simulink library "tqd"  (R2021b)
settings: Solver=VariableStepAuto  StartTime=0.0  StopTime=10.0  RelTol=1e-3
undefined symbols (not defined in the file or in its folder): ATQD_AccelLimitInRange_X_rpm, ATQD_AccelLimitInRange_Y_Nm, ATQD_AccelLimitOvrKi_X_Nm, ATQD_AccelLimitOvrKp_X_Nm, ATQD_BOSMapD_X_rpm, ATQD_BOSMapD_Y_pct, ATQD_BOSMapR_X_rpm, ATQD_BOSMapR_Y_pct, ATQD_HVBCurrSmooth_X_A, ATQD_LHMTqMapDLC_X_rpm, ATQD_LHMTqMapDLC_Y_pct, ATQD_LHMTqMapRLC_X_rpm, ATQD_LHMTqMapRLC_Y_pct, ATQD_NormalMapDLC_X_rpm, ATQD_NormalMapDLC_Y_pct, ATQD_NormalTqDecSR_X_rpm, ATQD_NormalTqDecSR_Y_Nm, ATQD_NormalTqIncSR_X_rpm, ATQD_NormalTqIncSR_Y_Nm, ATQD_OPDMapRLC_X_rpm, ATQD_OPDMapRLC_Y_pct, ATQD_RollRegTorReq_X_rpm, ATQD_RollRegTorReq_Y_enum, ATQD_VehSpdLimitInRange_X_rpm, ATQD_VehSpdLimitInRange_Y_Nm, ATQD_VehSpdLimitOvrKi_X_Nm, ATQD_VehSpdLimitOvrKp_X_Nm, EIGHT_INT, ENUM_BRAKEPEDAL_PRESSED, ENUM_BRAKEPEDAL_RELEASED, ENUM_COMBOKEY_DOWN, ENUM_COMBOKEY_M1, ENUM_COMBOKEY_M2, ENUM_COMBOKEY_NONE, ENUM_COMBOKEY_RKNEE, ENUM_COMBOKEY_STOPLV, ENUM_COMBOKEY_UP, ENUM_CP2VKNEEREQ_REQUEST, ENUM_CP2VNLVREQ_LEVEL1, ENUM_CP2VNLVREQ_LEVEL2, ENUM_CP2VNLVREQ_LOWER, ENUM_CP2VNLVREQ_STOPLV, ENUM_CP2VNLVREQ_UPPER, ENUM_CREEPIND_DISABLE, ENUM_CREEPIND_READY, ENUM_CREEPIND_RUNNING, ENUM_CREEPIND_WARNING, ENUM_DRIVELINERELEASE_RELEASE, ENUM_EBSTORQUERWQ_LIMIT, ENUM_EBSTORQUERWQ_TORQUE, ENUM_ECPVCUDRM_CONFORT, ENUM_ECPVCUDRM_ECO, ENUM_ECPVCUDRM_NORMAL, ENUM_ECPVCUDRM_NOTAVAILABLE, ENUM_EMTqModeDrvBrk_Accel, ENUM_EMTqModeDrvBrk_Brake, ENUM_EMTqModeDrvBrk_Coast, ENUM_ETC2ACTDRIVEDIR_BACKWARD, ENUM_ETC2ACTDRIVEDIR_FORWARD, ENUM_ETC2ACTDRIVEDIR_STILL ... (+341)
libraries: simulink x109, hcu_lib x67
(part 10 of 13)

== system tqd/TQD/Input_Convert/Input Signal Convert/Big Mike Combo V2 /Combo Key Detection/Function1 Alcohol Lock/Key8 ==
  VTQD_ComboKeyCMD_enum : Inport
  VTQD_ComboKeyEn_flg : Inport  Port=2
  VTQD_ComboKeyReset_flg : Inport  Port=3
  VTQD_ComboKey7_enum : Inport  Port=4
  AND : Logic  Inputs=4  AllPortsSameDT=off  OutDataTypeStr=boolean
  Constant1 : Constant  Value=KTQD_Function1Off8_enum
  Constant2 : Constant  Value=ENUM_COMBOKEY_NONE
  Constant3 : Constant  Value=ENUM_COMBOKEY_NONE
  Constant4 : Constant  Value=ENUM_COMBOKEY_NONE
  Data Type Conversion : DataTypeConversion  OutDataTypeStr=uint8
  Delay : Delay  DelayLength=1  InitialCondition=uint8(0)
      settings: AttributesFormatString=%<InitialCondition>
  Delay1 : Delay  DelayLength=1  InitialCondition=uint8(0)
      settings: AttributesFormatString=%<InitialCondition>
  Delay2 : Delay  DelayLength=1  InitialCondition=uint8(0)
      settings: AttributesFormatString=%<InitialCondition>
  Detect Change : simulink/Logic and Bit Operations/Detect Change  vinit=boolean(0)  OutDataTypeStr=boolean
  Detect Increase : simulink/Logic and Bit Operations/Detect Increase  vinit=boolean(0)  OutDataTypeStr=boolean
  Equal : RelationalOperator  Operator===  OutDataTypeStr=boolean  RndMeth=Simplest
  Equal1 : RelationalOperator  Operator=~=  OutDataTypeStr=boolean  RndMeth=Simplest
  Equal2 : RelationalOperator  Operator=~=  OutDataTypeStr=boolean  RndMeth=Simplest
  Equal3 : RelationalOperator  Operator===  OutDataTypeStr=boolean  RndMeth=Simplest
  If : If  NumInputs=2  IfExpression=u1 ~=0  ElseIfExpressions=u2 ~= 0
  Maintain : Subsystem  TreatAsAtomicUnit=on
  Merge : Merge  Inputs=3
  OR : Logic  Operator=OR  AllPortsSameDT=off  OutDataTypeStr=boolean
  Reset : Subsystem  TreatAsAtomicUnit=on
  Write : Subsystem  TreatAsAtomicUnit=on
  VTQD_ComboKey8_enum : Outport
  VTQD_Key8Pass_flg : Outport  Port=2
  wires:
  VTQD_ComboKeyEn_flg/1 -> [VTQD_ComboKeyEn_flg]
  VTQD_ComboKeyReset_flg/1 -> [VTQD_ComboKeyReset_flg]
  VTQD_ComboKeyCMD_enum/1 -> [VTQD_ComboKeyCMD_enum]
  Equal/1 -> [VTQD_Function1Off8Pass_flg]  "VTQD_Function1Off8Pass_flg"
  Constant1/1 -> Equal/2
  If/2 -> Write/Action
  Write/1(WriteCMD) -> Merge/2
  If/1 -> Reset/Action
  Detect Increase/1 -> OR/1
  AND/1 -> [VTQD_WriteComboCMD_flg]  "VTQD_WriteComboCMD_flg"
  [VTQD_ComboKeyCMD_enum] -> Write/1(Input)
  [VTQD_ComboKeyCMD_enum] -> Detect Change/1
  [VTQD_ResetComboKey_flg] -> If/1
  [VTQD_ComboKeyEn_flg] -> Detect Increase/1
  Detect Change/1 -> AND/1
  Maintain/1(KeepKey8) -> Merge/3
  Constant4/1 -> Equal1/2
  If/3 -> Maintain/Action
  Delay/1 -> Equal2/1
  Merge/1 -> Data Type Conversion/1
  Reset/1(ResetToZero) -> Merge/1
  Equal2/1 -> AND/3
  Constant2/1 -> Equal2/2
  Equal1/1 -> AND/2
  [VTQD_ComboKey7_enum] -> Delay/1
  [VTQD_ComboKeyReset_flg] -> OR/2
  [VTQD_ComboKeyCMD_enum] -> Equal1/1
  [VTQD_WriteComboCMD_flg] -> If/2
  OR/1 -> [VTQD_ResetComboKey_flg]  "VTQD_ResetComboKey_flg"
  VTQD_ComboKey7_enum/1 -> [VTQD_ComboKey7_enum]
  [VTQD_ComboKey8_enum] -> Delay1/1
  Constant3/1 -> Equal3/2
  Delay1/1 -> Equal3/1
  Equal3/1 -> AND/4
  [VTQD_Function1Off8Pass_flg] -> VTQD_Key8Pass_flg/1
  [VTQD_ComboKey8_enum] -> Equal/1
  [VTQD_ComboKey8_enum] -> VTQD_ComboKey8_enum/1
  [VTQD_ComboKey8_enum] -> Delay2/1
  Delay2/1 -> Maintain/1(Input)
  Data Type Conversion/1 -> [VTQD_ComboKey8_enum]  "VTQD_Function1Off8_enum"

== system tqd/TQD/Input_Convert/Input Signal Convert/Big Mike Combo V2 /Combo Key Detection/Function2 /Key1 ==
  VTQD_ComboKeyCMD_enum : Inport
  VTQD_ComboKeyEn_flg : Inport  Port=2
  VTQD_ComboKeyReset_flg : Inport  Port=3
  AND : Logic  Inputs=3  AllPortsSameDT=off  OutDataTypeStr=boolean
  Constant1 : Constant  Value=KTQD_Function2Off1_enum
  Constant2 : Constant  Value=ENUM_COMBOKEY_NONE
  Constant4 : Constant  Value=ENUM_COMBOKEY_NONE
  Data Type Conversion : DataTypeConversion  OutDataTypeStr=uint8
  Delay : Delay  DelayLength=1  InitialCondition=uint8(0)
      settings: AttributesFormatString=%<InitialCondition>
  Delay1 : Delay  DelayLength=1  InitialCondition=uint8(0)
      settings: AttributesFormatString=%<InitialCondition>
  Detect Change : simulink/Logic and Bit Operations/Detect Change  vinit=boolean(0)  OutDataTypeStr=boolean
  Detect Increase : simulink/Logic and Bit Operations/Detect Increase  vinit=boolean(0)  OutDataTypeStr=boolean
  Equal : RelationalOperator  Operator===  OutDataTypeStr=boolean  RndMeth=Simplest
  Equal1 : RelationalOperator  Operator=~=  OutDataTypeStr=boolean  RndMeth=Simplest
  Equal2 : RelationalOperator  Operator===  OutDataTypeStr=boolean  RndMeth=Simplest
  If : If  NumInputs=2  IfExpression=u1 ~=0  ElseIfExpressions=u2 ~= 0
  Maintain : Subsystem  TreatAsAtomicUnit=on
  Merge : Merge  Inputs=3
  OR : Logic  Operator=OR  AllPortsSameDT=off  OutDataTypeStr=boolean
  Reset : Subsystem  TreatAsAtomicUnit=on
  Write : Subsystem  TreatAsAtomicUnit=on
  VTQD_ComboKey1_enum : Outport
  VTQD_Key1Pass_flg : Outport  Port=2
  wires:
  Data Type Conversion/1 -> [VTQD_ComboKey1_enum]  "VTQD_Function2Off1_enum"
  Delay1/1 -> Maintain/1(Input)
  [VTQD_ComboKey1_enum] -> Delay1/1
  [VTQD_Key1Pass_flg] -> VTQD_Key1Pass_flg/1
  [VTQD_ComboKey1_enum] -> VTQD_ComboKey1_enum/1
  VTQD_ComboKeyEn_flg/1 -> [VTQD_ComboKeyEn_flg]
  VTQD_ComboKeyReset_flg/1 -> [VTQD_ComboKeyReset_flg]
  VTQD_ComboKeyCMD_enum/1 -> [VTQD_ComboKeyCMD_enum]
  Equal/1 -> [VTQD_Key1Pass_flg]  "VTQD_Function2Off1Pass_flg"
  Constant1/1 -> Equal/2
  [VTQD_ComboKey1_enum] -> Equal/1
  If/2 -> Write/Action
  Write/1(WriteCMD) -> Merge/2
  If/1 -> Reset/Action
  Detect Increase/1 -> OR/1
  AND/1 -> [VTQD_WriteComboCMD_flg]  "VTQD_WriteComboCMD_flg"
  [VTQD_ComboKeyCMD_enum] -> Write/1(Input)
  [VTQD_ComboKeyCMD_enum] -> Detect Change/1
  [VTQD_ResetComboKey_flg] -> If/1
  [VTQD_ComboKeyEn_flg] -> Detect Increase/1
  Detect Change/1 -> AND/1
  Maintain/1(KeepKey1) -> Merge/3
  Constant4/1 -> Equal1/2
  If/3 -> Maintain/Action
  Delay/1 -> Equal2/1
  Merge/1 -> Data Type Conversion/1
  Reset/1(ResetToZero) -> Merge/1
  Equal2/1 -> AND/3
  Constant2/1 -> Equal2/2
  Equal1/1 -> AND/2
  [VTQD_ComboKey1_enum] -> Delay/1
  [VTQD_ComboKeyReset_flg] -> OR/2
  [VTQD_ComboKeyCMD_enum] -> Equal1/1
  [VTQD_WriteComboCMD_flg] -> If/2
  OR/1 -> [VTQD_ResetComboKey_flg]  "VTQD_ResetComboKey_flg"

== system tqd/TQD/Input_Convert/Input Signal Convert/Big Mike Combo V2 /Combo Key Detection/Function2 /Key2 ==
  VTQD_ComboKeyCMD_enum : Inport
  VTQD_ComboKeyEn_flg : Inport  Port=2
  VTQD_ComboKeyReset_flg : Inport  Port=3
  VTQD_ComboKey1_enum : Inport  Port=4
  AND : Logic  Inputs=4  AllPortsSameDT=off  OutDataTypeStr=boolean
  Constant1 : Constant  Value=KTQD_Function2Off2_enum
  Constant2 : Constant  Value=ENUM_COMBOKEY_NONE
  Constant3 : Constant  Value=ENUM_COMBOKEY_NONE
  Constant4 : Constant  Value=ENUM_COMBOKEY_NONE  OutDataTypeStr=uint8
  Data Type Conversion : DataTypeConversion  OutDataTypeStr=uint8
  Delay : Delay  DelayLength=1  InitialCondition=uint8(0)
      settings: AttributesFormatString=%<InitialCondition>
  Delay1 : Delay  DelayLength=1  InitialCondition=uint8(0)
      settings: AttributesFormatString=%<InitialCondition>
  Delay2 : Delay  DelayLength=1  InitialCondition=uint8(0)
      settings: AttributesFormatString=%<InitialCondition>
  Detect Change : simulink/Logic and Bit Operations/Detect Change  vinit=boolean(0)  OutDataTypeStr=boolean
  Detect Increase : simulink/Logic and Bit Operations/Detect Increase  vinit=boolean(0)  OutDataTypeStr=boolean
  Equal : RelationalOperator  Operator===  OutDataTypeStr=boolean  RndMeth=Simplest
  Equal1 : RelationalOperator  Operator=~=  OutDataTypeStr=boolean  RndMeth=Simplest
  Equal2 : RelationalOperator  Operator=~=  OutDataTypeStr=boolean  RndMeth=Simplest
  Equal3 : RelationalOperator  Operator===  OutDataTypeStr=boolean  RndMeth=Simplest
  If : If  NumInputs=2  IfExpression=u1 ~=0  ElseIfExpressions=u2 ~= 0
  Maintain : Subsystem  TreatAsAtomicUnit=on
  Merge : Merge  Inputs=3
  OR : Logic  Operator=OR  AllPortsSameDT=off  OutDataTypeStr=boolean
  Reset : Subsystem  TreatAsAtomicUnit=on
  Write : Subsystem  TreatAsAtomicUnit=on
  VTQD_ComboKey2_enum : Outport
  VTQD_Key2Pass_flg : Outport  Port=2
  wires:
  Data Type Conversion/1 -> [VTQD_ComboKey2_enum]  "VTQD_Function2Off2_enum"
  [VTQD_ComboKey2_enum] -> Delay2/1
  Delay2/1 -> Maintain/1(Input)
  Equal3/1 -> AND/4
  Delay1/1 -> Equal3/1
  Constant3/1 -> Equal3/2
  [VTQD_ComboKey2_enum] -> Delay1/1
  VTQD_ComboKey1_enum/1 -> [VTQD_ComboKey1_enum]
  OR/1 -> [VTQD_ResetComboKey_flg]  "VTQD_ResetComboKey_flg"
  [VTQD_WriteComboCMD_flg] -> If/2
  [VTQD_ComboKeyCMD_enum] -> Equal1/1
  [VTQD_ComboKeyReset_flg] -> OR/2
  [VTQD_ComboKey1_enum] -> Delay/1
  Equal1/1 -> AND/2
  Constant2/1 -> Equal2/2
  Equal2/1 -> AND/3
  Reset/1(ResetToZero) -> Merge/1
  Merge/1 -> Data Type Conversion/1
  Delay/1 -> Equal2/1
  If/3 -> Maintain/Action
  Constant4/1 -> Equal1/2
  Maintain/1(KeepKey2) -> Merge/3
  Detect Change/1 -> AND/1
  [VTQD_ComboKeyEn_flg] -> Detect Increase/1
  [VTQD_ResetComboKey_flg] -> If/1
  [VTQD_ComboKeyCMD_enum] -> Detect Change/1
  [VTQD_ComboKeyCMD_enum] -> Write/1(Input)
  AND/1 -> [VTQD_WriteComboCMD_flg]  "VTQD_WriteComboCMD_flg"
  Detect Increase/1 -> OR/1
  If/1 -> Reset/Action
  Write/1(WriteCMD) -> Merge/2
  If/2 -> Write/Action
  [VTQD_ComboKey2_enum] -> Equal/1
  Constant1/1 -> Equal/2
  Equal/1 -> [VTQD_Key2Pass_flg]  "VTQD_Function2Off2Pass_flg"
  VTQD_ComboKeyCMD_enum/1 -> [VTQD_ComboKeyCMD_enum]
  VTQD_ComboKeyReset_flg/1 -> [VTQD_ComboKeyReset_flg]
  VTQD_ComboKeyEn_flg/1 -> [VTQD_ComboKeyEn_flg]
  [VTQD_ComboKey2_enum] -> VTQD_ComboKey2_enum/1
  [VTQD_Key2Pass_flg] -> VTQD_Key2Pass_flg/1

== system tqd/TQD/Input_Convert/Input Signal Convert/Big Mike Combo V2 /Combo Key Detection/Function2 /Key3 ==
  VTQD_ComboKeyCMD_enum : Inport
  VTQD_ComboKeyEn_flg : Inport  Port=2
  VTQD_ComboKeyReset_flg : Inport  Port=3
  VTQD_ComboKey2_enum : Inport  Port=4
  AND : Logic  Inputs=4  AllPortsSameDT=off  OutDataTypeStr=boolean
  Constant1 : Constant  Value=KTQD_Function2Off3_enum
  Constant2 : Constant  Value=ENUM_COMBOKEY_NONE
  Constant3 : Constant  Value=ENUM_COMBOKEY_NONE
  Constant4 : Constant  Value=ENUM_COMBOKEY_NONE
  Data Type Conversion : DataTypeConversion  OutDataTypeStr=uint8
  Delay : Delay  DelayLength=1  InitialCondition=uint8(0)
      settings: AttributesFormatString=%<InitialCondition>
  Delay1 : Delay  DelayLength=1  InitialCondition=uint8(0)
      settings: AttributesFormatString=%<InitialCondition>
  Delay2 : Delay  DelayLength=1  InitialCondition=uint8(0)
      settings: AttributesFormatString=%<InitialCondition>
  Detect Change : simulink/Logic and Bit Operations/Detect Change  vinit=boolean(0)  OutDataTypeStr=boolean
  Detect Increase : simulink/Logic and Bit Operations/Detect Increase  vinit=boolean(0)  OutDataTypeStr=boolean
  Equal : RelationalOperator  Operator===  OutDataTypeStr=boolean  RndMeth=Simplest
  Equal1 : RelationalOperator  Operator=~=  OutDataTypeStr=boolean  RndMeth=Simplest
  Equal2 : RelationalOperator  Operator=~=  OutDataTypeStr=boolean  RndMeth=Simplest
  Equal3 : RelationalOperator  Operator===  OutDataTypeStr=boolean  RndMeth=Simplest
  If : If  NumInputs=2  IfExpression=u1 ~=0  ElseIfExpressions=u2 ~= 0
  Maintain : Subsystem  TreatAsAtomicUnit=on
  Merge : Merge  Inputs=3
  OR : Logic  Operator=OR  AllPortsSameDT=off  OutDataTypeStr=boolean
  Reset : Subsystem  TreatAsAtomicUnit=on
  Write : Subsystem  TreatAsAtomicUnit=on
  VTQD_ComboKey3_enum : Outport
  VTQD_Key3Pass_flg : Outport  Port=2
  wires:
  Data Type Conversion/1 -> [VTQD_ComboKey3_enum]  "VTQD_Function2Off3_enum"
  [VTQD_ComboKey3_enum] -> Delay2/1
  Delay2/1 -> Maintain/1(Input)
  [VTQD_ComboKey3_enum] -> Delay1/1
  Constant3/1 -> Equal3/2
  Equal3/1 -> AND/4
  Delay1/1 -> Equal3/1
  [VTQD_Key3Pass_flg] -> VTQD_Key3Pass_flg/1
  [VTQD_ComboKey3_enum] -> Equal/1
  [VTQD_ComboKey3_enum] -> VTQD_ComboKey3_enum/1
  VTQD_ComboKeyEn_flg/1 -> [VTQD_ComboKeyEn_flg]
  VTQD_ComboKeyReset_flg/1 -> [VTQD_ComboKeyReset_flg]
  VTQD_ComboKeyCMD_enum/1 -> [VTQD_ComboKeyCMD_enum]
  Equal/1 -> [VTQD_Key3Pass_flg]  "VTQD_Function2Off3Pass_flg"
  Constant1/1 -> Equal/2
  If/2 -> Write/Action
  Write/1(WriteCMD) -> Merge/2
  If/1 -> Reset/Action
  Detect Increase/1 -> OR/1
  AND/1 -> [VTQD_WriteComboCMD_flg]  "VTQD_WriteComboCMD_flg"
  [VTQD_ComboKeyCMD_enum] -> Write/1(Input)
  [VTQD_ComboKeyCMD_enum] -> Detect Change/1
  [VTQD_ResetComboKey_flg] -> If/1
  [VTQD_ComboKeyEn_flg] -> Detect Increase/1
  Detect Change/1 -> AND/1
  Maintain/1(KeepKey3) -> Merge/3
  Constant4/1 -> Equal1/2
  If/3 -> Maintain/Action
  Delay/1 -> Equal2/1
  Merge/1 -> Data Type Conversion/1
  Reset/1(ResetToZero) -> Merge/1
  Equal2/1 -> AND/3
  Constant2/1 -> Equal2/2
  Equal1/1 -> AND/2
  [VTQD_ComboKey2_enum] -> Delay/1
  [VTQD_ComboKeyReset_flg] -> OR/2
  [VTQD_ComboKeyCMD_enum] -> Equal1/1
  [VTQD_WriteComboCMD_flg] -> If/2
  OR/1 -> [VTQD_ResetComboKey_flg]  "VTQD_ResetComboKey_flg"
  VTQD_ComboKey2_enum/1 -> [VTQD_ComboKey2_enum]

== system tqd/TQD/Input_Convert/Input Signal Convert/Big Mike Combo V2 /Combo Key Detection/Function2 /Key4 ==
  VTQD_ComboKeyCMD_enum : Inport
  VTQD_ComboKeyEn_flg : Inport  Port=2
  VTQD_ComboKeyReset_flg : Inport  Port=3
  VTQD_ComboKey3_enum : Inport  Port=4
  AND : Logic  Inputs=4  AllPortsSameDT=off  OutDataTypeStr=boolean
  Constant1 : Constant  Value=KTQD_Function2Off4_enum
  Constant2 : Constant  Value=ENUM_COMBOKEY_NONE
  Constant3 : Constant  Value=ENUM_COMBOKEY_NONE
  Constant4 : Constant  Value=ENUM_COMBOKEY_NONE
  Data Type Conversion : DataTypeConversion  OutDataTypeStr=uint8
  Delay : Delay  DelayLength=1  InitialCondition=uint8(0)
      settings: AttributesFormatString=%<InitialCondition>
  Delay1 : Delay  DelayLength=1  InitialCondition=uint8(0)
      settings: AttributesFormatString=%<InitialCondition>
  Delay2 : Delay  DelayLength=1  InitialCondition=uint8(0)
      settings: AttributesFormatString=%<InitialCondition>
  Detect Change : simulink/Logic and Bit Operations/Detect Change  vinit=boolean(0)  OutDataTypeStr=boolean
  Detect Increase : simulink/Logic and Bit Operations/Detect Increase  vinit=boolean(0)  OutDataTypeStr=boolean
  Equal : RelationalOperator  Operator===  OutDataTypeStr=boolean  RndMeth=Simplest
  Equal1 : RelationalOperator  Operator=~=  OutDataTypeStr=boolean  RndMeth=Simplest
  Equal2 : RelationalOperator  Operator=~=  OutDataTypeStr=boolean  RndMeth=Simplest
  Equal3 : RelationalOperator  Operator===  OutDataTypeStr=boolean  RndMeth=Simplest
  If : If  NumInputs=2  IfExpression=u1 ~=0  ElseIfExpressions=u2 ~= 0
  Maintain : Subsystem  TreatAsAtomicUnit=on
  Merge : Merge  Inputs=3
  OR : Logic  Operator=OR  AllPortsSameDT=off  OutDataTypeStr=boolean
  Reset : Subsystem  TreatAsAtomicUnit=on
  Write : Subsystem  TreatAsAtomicUnit=on
  VTQD_ComboKey4_enum : Outport
  VTQD_Key4Pass_flg : Outport  Port=2
  wires:
  Data Type Conversion/1 -> [VTQD_ComboKey4_enum]  "VTQD_Function2Off4_enum"
  Delay2/1 -> Maintain/1(Input)
  [VTQD_ComboKey4_enum] -> Delay2/1
  [VTQD_ComboKey4_enum] -> VTQD_ComboKey4_enum/1
  [VTQD_Key4Pass_flg] -> VTQD_Key4Pass_flg/1
  Equal3/1 -> AND/4
  Delay1/1 -> Equal3/1
  Constant3/1 -> Equal3/2
  [VTQD_ComboKey4_enum] -> Delay1/1
  VTQD_ComboKey3_enum/1 -> [VTQD_ComboKey3_enum]
  OR/1 -> [VTQD_ResetComboKey_flg]  "VTQD_ResetComboKey_flg"
  [VTQD_WriteComboCMD_flg] -> If/2
  [VTQD_ComboKeyCMD_enum] -> Equal1/1
  [VTQD_ComboKeyReset_flg] -> OR/2
  [VTQD_ComboKey3_enum] -> Delay/1
  Equal1/1 -> AND/2
  Constant2/1 -> Equal2/2
  Equal2/1 -> AND/3
  Reset/1(ResetToZero) -> Merge/1
  Merge/1 -> Data Type Conversion/1
  Delay/1 -> Equal2/1
  If/3 -> Maintain/Action
  Constant4/1 -> Equal1/2
  Maintain/1(KeepKey4) -> Merge/3
  Detect Change/1 -> AND/1
  [VTQD_ComboKeyEn_flg] -> Detect Increase/1
  [VTQD_ResetComboKey_flg] -> If/1
  [VTQD_ComboKeyCMD_enum] -> Detect Change/1
  [VTQD_ComboKeyCMD_enum] -> Write/1(Input)
  AND/1 -> [VTQD_WriteComboCMD_flg]  "VTQD_WriteComboCMD_flg"
  Detect Increase/1 -> OR/1
  If/1 -> Reset/Action
  Write/1(WriteCMD) -> Merge/2
  If/2 -> Write/Action
  Constant1/1 -> Equal/2
  Equal/1 -> [VTQD_Key4Pass_flg]  "VTQD_Function2Off4Pass_flg"
  VTQD_ComboKeyCMD_enum/1 -> [VTQD_ComboKeyCMD_enum]
  VTQD_ComboKeyReset_flg/1 -> [VTQD_ComboKeyReset_flg]
  VTQD_ComboKeyEn_flg/1 -> [VTQD_ComboKeyEn_flg]
  [VTQD_ComboKey4_enum] -> Equal/1

== system tqd/TQD/Input_Convert/Input Signal Convert/Big Mike Combo V2 /Combo Key Detection/Function2 /Key5 ==
  VTQD_ComboKeyCMD_enum : Inport
  VTQD_ComboKeyEn_flg : Inport  Port=2
  VTQD_ComboKeyReset_flg : Inport  Port=3
  VTQD_ComboKey4_enum : Inport  Port=4
  AND : Logic  Inputs=4  AllPortsSameDT=off  OutDataTypeStr=boolean
  Constant1 : Constant  Value=KTQD_Function2Off5_enum
  Constant2 : Constant  Value=ENUM_COMBOKEY_NONE
  Constant3 : Constant  Value=ENUM_COMBOKEY_NONE
  Constant4 : Constant  Value=ENUM_COMBOKEY_NONE
  Data Type Conversion : DataTypeConversion  OutDataTypeStr=uint8
  Delay : Delay  DelayLength=1  InitialCondition=uint8(0)
      settings: AttributesFormatString=%<InitialCondition>
  Delay1 : Delay  DelayLength=1  InitialCondition=uint8(0)
      settings: AttributesFormatString=%<InitialCondition>
  Delay2 : Delay  DelayLength=1  InitialCondition=uint8(0)
      settings: AttributesFormatString=%<InitialCondition>
  Detect Change : simulink/Logic and Bit Operations/Detect Change  vinit=boolean(0)  OutDataTypeStr=boolean
  Detect Increase : simulink/Logic and Bit Operations/Detect Increase  vinit=boolean(0)  OutDataTypeStr=boolean
  Equal : RelationalOperator  Operator===  OutDataTypeStr=boolean  RndMeth=Simplest
  Equal1 : RelationalOperator  Operator=~=  OutDataTypeStr=boolean  RndMeth=Simplest
  Equal2 : RelationalOperator  Operator=~=  OutDataTypeStr=boolean  RndMeth=Simplest
  Equal3 : RelationalOperator  Operator===  OutDataTypeStr=boolean  RndMeth=Simplest
  If : If  NumInputs=2  IfExpression=u1 ~=0  ElseIfExpressions=u2 ~= 0
  Maintain : Subsystem  TreatAsAtomicUnit=on
  Merge : Merge  Inputs=3
  OR : Logic  Operator=OR  AllPortsSameDT=off  OutDataTypeStr=boolean
  Reset : Subsystem  TreatAsAtomicUnit=on
  Write : Subsystem  TreatAsAtomicUnit=on
  VTQD_ComboKey5_enum : Outport
  VTQD_Key5Pass_flg : Outport  Port=2
  wires:
  Data Type Conversion/1 -> [VTQD_ComboKey5_enum]  "VTQD_Function2Off5_enum"
  Delay2/1 -> Maintain/1(Input)
  [VTQD_ComboKey5_enum] -> Delay2/1
  [VTQD_ComboKey5_enum] -> VTQD_ComboKey5_enum/1
  [VTQD_ComboKey5_enum] -> Equal/1
  VTQD_ComboKeyEn_flg/1 -> [VTQD_ComboKeyEn_flg]
  VTQD_ComboKeyReset_flg/1 -> [VTQD_ComboKeyReset_flg]
  VTQD_ComboKeyCMD_enum/1 -> [VTQD_ComboKeyCMD_enum]
  Equal/1 -> [VTQD_Key5Pass_flg]  "VTQD_Function2Off5Pass_flg"
  Constant1/1 -> Equal/2
  If/2 -> Write/Action
  Write/1(WriteCMD) -> Merge/2
  If/1 -> Reset/Action
  Detect Increase/1 -> OR/1
  AND/1 -> [VTQD_WriteComboCMD_flg]  "VTQD_WriteComboCMD_flg"
  [VTQD_ComboKeyCMD_enum] -> Write/1(Input)
  [VTQD_ComboKeyCMD_enum] -> Detect Change/1
  [VTQD_ResetComboKey_flg] -> If/1
  [VTQD_ComboKeyEn_flg] -> Detect Increase/1
  Detect Change/1 -> AND/1
  Maintain/1(KeepKey5) -> Merge/3
  Constant4/1 -> Equal1/2
  If/3 -> Maintain/Action
  Delay/1 -> Equal2/1
  Merge/1 -> Data Type Conversion/1
  Reset/1(ResetToZero) -> Merge/1
  Equal2/1 -> AND/3
  Constant2/1 -> Equal2/2
  Equal1/1 -> AND/2
  [VTQD_ComboKey4_enum] -> Delay/1
  [VTQD_ComboKeyReset_flg] -> OR/2
  [VTQD_ComboKeyCMD_enum] -> Equal1/1
  [VTQD_WriteComboCMD_flg] -> If/2
  OR/1 -> [VTQD_ResetComboKey_flg]  "VTQD_ResetComboKey_flg"
  VTQD_ComboKey4_enum/1 -> [VTQD_ComboKey4_enum]
  [VTQD_ComboKey5_enum] -> Delay1/1
  Constant3/1 -> Equal3/2
  Delay1/1 -> Equal3/1
  Equal3/1 -> AND/4
  [VTQD_Key5Pass_flg] -> VTQD_Key5Pass_flg/1

== system tqd/TQD/Input_Convert/Input Signal Convert/Big Mike Combo V2 /Combo Key Detection/Function2 /Key6 ==
  VTQD_ComboKeyCMD_enum : Inport
  VTQD_ComboKeyEn_flg : Inport  Port=2
  VTQD_ComboKeyReset_flg : Inport  Port=3
  VTQD_ComboKey5_enum : Inport  Port=4
  AND : Logic  Inputs=4  AllPortsSameDT=off  OutDataTypeStr=boolean
  Constant1 : Constant  Value=KTQD_Function2Off6_enum
  Constant2 : Constant  Value=ENUM_COMBOKEY_NONE
  Constant3 : Constant  Value=ENUM_COMBOKEY_NONE
  Constant4 : Constant  Value=ENUM_COMBOKEY_NONE
  Data Type Conversion : DataTypeConversion  OutDataTypeStr=uint8
  Delay : Delay  DelayLength=1  InitialCondition=uint8(0)
      settings: AttributesFormatString=%<InitialCondition>
  Delay1 : Delay  DelayLength=1  InitialCondition=uint8(0)
      settings: AttributesFormatString=%<InitialCondition>
  Delay2 : Delay  DelayLength=1  InitialCondition=uint8(0)
      settings: AttributesFormatString=%<InitialCondition>
  Detect Change : simulink/Logic and Bit Operations/Detect Change  vinit=boolean(0)  OutDataTypeStr=boolean
  Detect Increase : simulink/Logic and Bit Operations/Detect Increase  vinit=boolean(0)  OutDataTypeStr=boolean
  Equal : RelationalOperator  Operator===  OutDataTypeStr=boolean  RndMeth=Simplest
  Equal1 : RelationalOperator  Operator=~=  OutDataTypeStr=boolean  RndMeth=Simplest
  Equal2 : RelationalOperator  Operator=~=  OutDataTypeStr=boolean  RndMeth=Simplest
  Equal3 : RelationalOperator  Operator===  OutDataTypeStr=boolean  RndMeth=Simplest
  If : If  NumInputs=2  IfExpression=u1 ~=0  ElseIfExpressions=u2 ~= 0
  Maintain : Subsystem  TreatAsAtomicUnit=on
  Merge : Merge  Inputs=3
  OR : Logic  Operator=OR  AllPortsSameDT=off  OutDataTypeStr=boolean
  Reset : Subsystem  TreatAsAtomicUnit=on
  Write : Subsystem  TreatAsAtomicUnit=on
  VTQD_ComboKey6_enum : Outport
  VTQD_Key6Pass_flg : Outport  Port=2
  wires:
  Data Type Conversion/1 -> [VTQD_ComboKey6_enum]  "VTQD_Function2Off6_enum"
  [VTQD_ComboKey6_enum] -> Delay2/1
  Delay2/1 -> Maintain/1(Input)
  [VTQD_Key6Pass_flg] -> VTQD_Key6Pass_flg/1
  Equal3/1 -> AND/4
  Delay1/1 -> Equal3/1
  Constant3/1 -> Equal3/2
  [VTQD_ComboKey6_enum] -> Delay1/1
  VTQD_ComboKey5_enum/1 -> [VTQD_ComboKey5_enum]
  OR/1 -> [VTQD_ResetComboKey_flg]  "VTQD_ResetComboKey_flg"
  [VTQD_WriteComboCMD_flg] -> If/2
  [VTQD_ComboKeyCMD_enum] -> Equal1/1
  [VTQD_ComboKeyReset_flg] -> OR/2
  [VTQD_ComboKey5_enum] -> Delay/1
  Equal1/1 -> AND/2
  Constant2/1 -> Equal2/2
  Equal2/1 -> AND/3
  Reset/1(ResetToZero) -> Merge/1
  Merge/1 -> Data Type Conversion/1
  Delay/1 -> Equal2/1
  If/3 -> Maintain/Action
  Constant4/1 -> Equal1/2
  Maintain/1(KeepKey6) -> Merge/3
  Detect Change/1 -> AND/1
  [VTQD_ComboKeyEn_flg] -> Detect Increase/1
  [VTQD_ResetComboKey_flg] -> If/1
  [VTQD_ComboKeyCMD_enum] -> Detect Change/1
  [VTQD_ComboKeyCMD_enum] -> Write/1(Input)
  AND/1 -> [VTQD_WriteComboCMD_flg]  "VTQD_WriteComboCMD_flg"
  Detect Increase/1 -> OR/1
  If/1 -> Reset/Action
  Write/1(WriteCMD) -> Merge/2
  If/2 -> Write/Action
  Constant1/1 -> Equal/2
  Equal/1 -> [VTQD_Key6Pass_flg]  "VTQD_Function2Off6Pass_flg"
  VTQD_ComboKeyCMD_enum/1 -> [VTQD_ComboKeyCMD_enum]
  VTQD_ComboKeyReset_flg/1 -> [VTQD_ComboKeyReset_flg]
  VTQD_ComboKeyEn_flg/1 -> [VTQD_ComboKeyEn_flg]
  [VTQD_ComboKey6_enum] -> Equal/1
  [VTQD_ComboKey6_enum] -> VTQD_ComboKey6_enum/1

== system tqd/TQD/Input_Convert/Input Signal Convert/Big Mike Combo V2 /Combo Key Detection/Function2 /Key7 ==
  VTQD_ComboKeyCMD_enum : Inport
  VTQD_ComboKeyEn_flg : Inport  Port=2
  VTQD_ComboKeyReset_flg : Inport  Port=3
  VTQD_ComboKey6_enum : Inport  Port=4
  AND : Logic  Inputs=4  AllPortsSameDT=off  OutDataTypeStr=boolean
  Constant1 : Constant  Value=KTQD_Function2Off7_enum
  Constant2 : Constant  Value=ENUM_COMBOKEY_NONE  OutDataTypeStr=uint8
  Constant3 : Constant  Value=ENUM_COMBOKEY_NONE
  Constant4 : Constant  Value=ENUM_COMBOKEY_NONE  OutDataTypeStr=uint8
  Data Type Conversion : DataTypeConversion  OutDataTypeStr=uint8
  Delay : Delay  DelayLength=1  InitialCondition=uint8(0)
      settings: AttributesFormatString=%<InitialCondition>
  Delay1 : Delay  DelayLength=1  InitialCondition=uint8(0)
      settings: AttributesFormatString=%<InitialCondition>
  Delay2 : Delay  DelayLength=1  InitialCondition=uint8(0)
      settings: AttributesFormatString=%<InitialCondition>
  Detect Change : simulink/Logic and Bit Operations/Detect Change  vinit=boolean(0)  OutDataTypeStr=boolean
  Detect Increase : simulink/Logic and Bit Operations/Detect Increase  vinit=boolean(0)  OutDataTypeStr=boolean
  Equal : RelationalOperator  Operator===  OutDataTypeStr=boolean  RndMeth=Simplest
  Equal1 : RelationalOperator  Operator=~=  OutDataTypeStr=boolean  RndMeth=Simplest
  Equal2 : RelationalOperator  Operator=~=  OutDataTypeStr=boolean  RndMeth=Simplest
  Equal3 : RelationalOperator  Operator===  OutDataTypeStr=boolean  RndMeth=Simplest
  If : If  NumInputs=2  IfExpression=u1 ~=0  ElseIfExpressions=u2 ~= 0
  Maintain : Subsystem  TreatAsAtomicUnit=on
  Merge : Merge  Inputs=3
  OR : Logic  Operator=OR  AllPortsSameDT=off  OutDataTypeStr=boolean
  Reset : Subsystem  TreatAsAtomicUnit=on
  Write : Subsystem  TreatAsAtomicUnit=on
  VTQD_ComboKey7_enum : Outport
  VTQD_Key7Pass_flg : Outport  Port=2
  wires:
  Data Type Conversion/1 -> [VTQD_ComboKey7_enum]  "VTQD_Function2Off7_enum"
  Delay2/1 -> Maintain/1(Input)
  [VTQD_ComboKey7_enum] -> Delay2/1
  [VTQD_ComboKey7_enum] -> VTQD_ComboKey7_enum/1
  [VTQD_ComboKey7_enum] -> Equal/1
  VTQD_ComboKeyEn_flg/1 -> [VTQD_ComboKeyEn_flg]
  VTQD_ComboKeyReset_flg/1 -> [VTQD_ComboKeyReset_flg]
  VTQD_ComboKeyCMD_enum/1 -> [VTQD_ComboKeyCMD_enum]
  Equal/1 -> [VTQD_Key7Pass_flg]  "VTQD_Function2Off7Pass_flg"
  Constant1/1 -> Equal/2
  If/2 -> Write/Action
  Write/1(WriteCMD) -> Merge/2
  If/1 -> Reset/Action
  Detect Increase/1 -> OR/1
  AND/1 -> [VTQD_WriteComboCMD_flg]  "VTQD_WriteComboCMD_flg"
  [VTQD_ComboKeyCMD_enum] -> Write/1(Input)
  [VTQD_ComboKeyCMD_enum] -> Detect Change/1
  [VTQD_ResetComboKey_flg] -> If/1
  [VTQD_ComboKeyEn_flg] -> Detect Increase/1
  Detect Change/1 -> AND/1
  Maintain/1(KeepKey7) -> Merge/3
  Constant4/1 -> Equal1/2
  If/3 -> Maintain/Action
  Delay/1 -> Equal2/1
  Merge/1 -> Data Type Conversion/1
  Reset/1(ResetToZero) -> Merge/1
  Equal2/1 -> AND/3
  Constant2/1 -> Equal2/2
  Equal1/1 -> AND/2
  [VTQD_ComboKey6_enum] -> Delay/1
  [VTQD_ComboKeyReset_flg] -> OR/2
  [VTQD_ComboKeyCMD_enum] -> Equal1/1
  [VTQD_WriteComboCMD_flg] -> If/2
  OR/1 -> [VTQD_ResetComboKey_flg]  "VTQD_ResetComboKey_flg"
  VTQD_ComboKey6_enum/1 -> [VTQD_ComboKey6_enum]
  [VTQD_ComboKey7_enum] -> Delay1/1
  Constant3/1 -> Equal3/2
  Delay1/1 -> Equal3/1
  Equal3/1 -> AND/4
  [VTQD_Key7Pass_flg] -> VTQD_Key7Pass_flg/1

== system tqd/TQD/Input_Convert/Input Signal Convert/Big Mike Combo V2 /Combo Key Detection/Function2 /Key8 ==
  VTQD_ComboKeyCMD_enum : Inport
  VTQD_ComboKeyEn_flg : Inport  Port=2
  VTQD_ComboKeyReset_flg : Inport  Port=3
  VTQD_ComboKey7_enum : Inport  Port=4
  AND : Logic  Inputs=4  AllPortsSameDT=off  OutDataTypeStr=boolean
  Constant1 : Constant  Value=KTQD_Function2Off8_enum
  Constant2 : Constant  Value=ENUM_COMBOKEY_NONE
  Constant3 : Constant  Value=ENUM_COMBOKEY_NONE
  Constant4 : Constant  Value=ENUM_COMBOKEY_NONE
  Data Type Conversion : DataTypeConversion  OutDataTypeStr=uint8
  Delay : Delay  DelayLength=1  InitialCondition=uint8(0)
      settings: AttributesFormatString=%<InitialCondition>
  Delay1 : Delay  DelayLength=1  InitialCondition=uint8(0)
      settings: AttributesFormatString=%<InitialCondition>
  Delay2 : Delay  DelayLength=1  InitialCondition=uint8(0)
      settings: AttributesFormatString=%<InitialCondition>
  Detect Change : simulink/Logic and Bit Operations/Detect Change  vinit=boolean(0)  OutDataTypeStr=boolean
  Detect Increase : simulink/Logic and Bit Operations/Detect Increase  vinit=boolean(0)  OutDataTypeStr=boolean
  Equal : RelationalOperator  Operator===  OutDataTypeStr=boolean  RndMeth=Simplest
  Equal1 : RelationalOperator  Operator=~=  OutDataTypeStr=boolean  RndMeth=Simplest
  Equal2 : RelationalOperator  Operator=~=  OutDataTypeStr=boolean  RndMeth=Simplest
  Equal3 : RelationalOperator  Operator===  OutDataTypeStr=boolean  RndMeth=Simplest
  If : If  NumInputs=2  IfExpression=u1 ~=0  ElseIfExpressions=u2 ~= 0
  Maintain : Subsystem  TreatAsAtomicUnit=on
  Merge : Merge  Inputs=3
  OR : Logic  Operator=OR  AllPortsSameDT=off  OutDataTypeStr=boolean
  Reset : Subsystem  TreatAsAtomicUnit=on
  Write : Subsystem  TreatAsAtomicUnit=on
  VTQD_ComboKey8_enum : Outport
  VTQD_Key8Pass_flg : Outport  Port=2
  wires:
  Data Type Conversion/1 -> [VTQD_ComboKey8_enum]  "VTQD_Function2Off8_enum"
  Delay2/1 -> Maintain/1(Input)
  [VTQD_ComboKey8_enum] -> Delay2/1
  [VTQD_ComboKey8_enum] -> VTQD_ComboKey8_enum/1
  [VTQD_ComboKey8_enum] -> Equal/1
  [VTQD_Key8Pass_flg] -> VTQD_Key8Pass_flg/1
  Equal3/1 -> AND/4
  Delay1/1 -> Equal3/1
  Constant3/1 -> Equal3/2
  [VTQD_ComboKey8_enum] -> Delay1/1
  VTQD_ComboKey7_enum/1 -> [VTQD_ComboKey7_enum]
  OR/1 -> [VTQD_ResetComboKey_flg]  "VTQD_ResetComboKey_flg"
  [VTQD_WriteComboCMD_flg] -> If/2
  [VTQD_ComboKeyCMD_enum] -> Equal1/1
  [VTQD_ComboKeyReset_flg] -> OR/2
  [VTQD_ComboKey7_enum] -> Delay/1
  Equal1/1 -> AND/2
  Constant2/1 -> Equal2/2
  Equal2/1 -> AND/3
  Reset/1(ResetToZero) -> Merge/1
  Merge/1 -> Data Type Conversion/1
  Delay/1 -> Equal2/1
  If/3 -> Maintain/Action
  Constant4/1 -> Equal1/2
  Maintain/1(KeepKey8) -> Merge/3
  Detect Change/1 -> AND/1
  [VTQD_ComboKeyEn_flg] -> Detect Increase/1
  [VTQD_ResetComboKey_flg] -> If/1
  [VTQD_ComboKeyCMD_enum] -> Detect Change/1
  [VTQD_ComboKeyCMD_enum] -> Write/1(Input)
  AND/1 -> [VTQD_WriteComboCMD_flg]  "VTQD_WriteComboCMD_flg"
  Detect Increase/1 -> OR/1
  If/1 -> Reset/Action
  Write/1(WriteCMD) -> Merge/2
  If/2 -> Write/Action
  Constant1/1 -> Equal/2
  Equal/1 -> [VTQD_Key8Pass_flg]  "VTQD_Function2Off8Pass_flg"
  VTQD_ComboKeyCMD_enum/1 -> [VTQD_ComboKeyCMD_enum]
  VTQD_ComboKeyReset_flg/1 -> [VTQD_ComboKeyReset_flg]
  VTQD_ComboKeyEn_flg/1 -> [VTQD_ComboKeyEn_flg]

== system tqd/TQD/Input_Convert/Input Signal Convert/Big Mike Combo V2 /Combo Key Detection/Function3/Key1 ==
  VTQD_ComboKeyCMD_enum : Inport
  VTQD_ComboKeyEn_flg : Inport  Port=2
  VTQD_ComboKeyReset_flg : Inport  Port=3
  AND : Logic  Inputs=3  AllPortsSameDT=off  OutDataTypeStr=boolean
  Constant1 : Constant  Value=KTQD_Function3Off1_enum
  Constant2 : Constant  Value=ENUM_COMBOKEY_NONE
  Constant4 : Constant  Value=ENUM_COMBOKEY_NONE
  Data Type Conversion : DataTypeConversion  OutDataTypeStr=uint8
  Delay : Delay  DelayLength=1  InitialCondition=uint8(0)
      settings: AttributesFormatString=%<InitialCondition>
  Delay1 : Delay  DelayLength=1  InitialCondition=uint8(0)
      settings: AttributesFormatString=%<InitialCondition>
  Detect Change : simulink/Logic and Bit Operations/Detect Change  vinit=boolean(0)  OutDataTypeStr=boolean
  Detect Increase : simulink/Logic and Bit Operations/Detect Increase  vinit=boolean(0)  OutDataTypeStr=boolean
  Equal : RelationalOperator  Operator===  OutDataTypeStr=boolean  RndMeth=Simplest
  Equal1 : RelationalOperator  Operator=~=  OutDataTypeStr=boolean  RndMeth=Simplest
  Equal2 : RelationalOperator  Operator===  OutDataTypeStr=boolean  RndMeth=Simplest
  If : If  NumInputs=2  IfExpression=u1 ~=0  ElseIfExpressions=u2 ~= 0
  Maintain : Subsystem  TreatAsAtomicUnit=on
  Merge : Merge  Inputs=3
  OR : Logic  Operator=OR  AllPortsSameDT=off  OutDataTypeStr=boolean
  Reset : Subsystem  TreatAsAtomicUnit=on
  Write : Subsystem  TreatAsAtomicUnit=on
  VTQD_ComboKey1_enum : Outport
  VTQD_Key1Pass_flg : Outport  Port=2
  wires:
  OR/1 -> [VTQD_ResetComboKey_flg]  "VTQD_ResetComboKey_flg"
  [VTQD_WriteComboCMD_flg] -> If/2
  [VTQD_ComboKeyCMD_enum] -> Equal1/1
  [VTQD_ComboKeyReset_flg] -> OR/2
  [VTQD_ComboKey1_enum] -> Delay/1
  Equal1/1 -> AND/2
  Constant2/1 -> Equal2/2
  Equal2/1 -> AND/3
  Reset/1(ResetToZero) -> Merge/1
  Merge/1 -> Data Type Conversion/1
  Delay/1 -> Equal2/1
  If/3 -> Maintain/Action
  Constant4/1 -> Equal1/2
  Maintain/1(KeepKey1) -> Merge/3
  Detect Change/1 -> AND/1
  [VTQD_ComboKeyEn_flg] -> Detect Increase/1
  [VTQD_ResetComboKey_flg] -> If/1
  [VTQD_ComboKeyCMD_enum] -> Detect Change/1
  [VTQD_ComboKeyCMD_enum] -> Write/1(Input)
  AND/1 -> [VTQD_WriteComboCMD_flg]  "VTQD_WriteComboCMD_flg"
  Detect Increase/1 -> OR/1
  If/1 -> Reset/Action
  Write/1(WriteCMD) -> Merge/2
  If/2 -> Write/Action
  [VTQD_ComboKey1_enum] -> Equal/1
  Constant1/1 -> Equal/2
  Equal/1 -> [VTQD_Key1Pass_flg]  "VTQD_Function3Off1Pass_flg"
  VTQD_ComboKeyCMD_enum/1 -> [VTQD_ComboKeyCMD_enum]
  VTQD_ComboKeyReset_flg/1 -> [VTQD_ComboKeyReset_flg]
  VTQD_ComboKeyEn_flg/1 -> [VTQD_ComboKeyEn_flg]
  [VTQD_ComboKey1_enum] -> VTQD_ComboKey1_enum/1
  [VTQD_Key1Pass_flg] -> VTQD_Key1Pass_flg/1
  [VTQD_ComboKey1_enum] -> Delay1/1
  Delay1/1 -> Maintain/1(Input)
  Data Type Conversion/1 -> [VTQD_ComboKey1_enum]  "VTQD_Function3Off1_enum"

== system tqd/TQD/Input_Convert/Input Signal Convert/Big Mike Combo V2 /Combo Key Detection/Function3/Key2 ==
  VTQD_ComboKeyCMD_enum : Inport
  VTQD_ComboKeyEn_flg : Inport  Port=2
  VTQD_ComboKeyReset_flg : Inport  Port=3
  VTQD_ComboKey1_enum : Inport  Port=4
  AND : Logic  Inputs=4  AllPortsSameDT=off  OutDataTypeStr=boolean
  Constant1 : Constant  Value=KTQD_Function3Off2_enum
  Constant2 : Constant  Value=ENUM_COMBOKEY_NONE
  Constant3 : Constant  Value=ENUM_COMBOKEY_NONE
  Constant4 : Constant  Value=ENUM_COMBOKEY_NONE  OutDataTypeStr=uint8
  Data Type Conversion : DataTypeConversion  OutDataTypeStr=uint8
  Delay : Delay  DelayLength=1  InitialCondition=uint8(0)
      settings: AttributesFormatString=%<InitialCondition>
  Delay1 : Delay  DelayLength=1  InitialCondition=uint8(0)
      settings: AttributesFormatString=%<InitialCondition>
  Delay2 : Delay  DelayLength=1  InitialCondition=uint8(0)
      settings: AttributesFormatString=%<InitialCondition>
  Detect Change : simulink/Logic and Bit Operations/Detect Change  vinit=boolean(0)  OutDataTypeStr=boolean
  Detect Increase : simulink/Logic and Bit Operations/Detect Increase  vinit=boolean(0)  OutDataTypeStr=boolean
  Equal : RelationalOperator  Operator===  OutDataTypeStr=boolean  RndMeth=Simplest
  Equal1 : RelationalOperator  Operator=~=  OutDataTypeStr=boolean  RndMeth=Simplest
  Equal2 : RelationalOperator  Operator=~=  OutDataTypeStr=boolean  RndMeth=Simplest
  Equal3 : RelationalOperator  Operator===  OutDataTypeStr=boolean  RndMeth=Simplest
  If : If  NumInputs=2  IfExpression=u1 ~=0  ElseIfExpressions=u2 ~= 0
  Maintain : Subsystem  TreatAsAtomicUnit=on
  Merge : Merge  Inputs=3
  OR : Logic  Operator=OR  AllPortsSameDT=off  OutDataTypeStr=boolean
  Reset : Subsystem  TreatAsAtomicUnit=on
  Write : Subsystem  TreatAsAtomicUnit=on
  VTQD_ComboKey2_enum : Outport
  VTQD_Key2Pass_flg : Outport  Port=2
  wires:
  [VTQD_Key2Pass_flg] -> VTQD_Key2Pass_flg/1
  [VTQD_ComboKey2_enum] -> VTQD_ComboKey2_enum/1
  VTQD_ComboKeyEn_flg/1 -> [VTQD_ComboKeyEn_flg]
  VTQD_ComboKeyReset_flg/1 -> [VTQD_ComboKeyReset_flg]
  VTQD_ComboKeyCMD_enum/1 -> [VTQD_ComboKeyCMD_enum]
  Equal/1 -> [VTQD_Key2Pass_flg]  "VTQD_Function3Off2Pass_flg"
  Constant1/1 -> Equal/2
  [VTQD_ComboKey2_enum] -> Equal/1
  If/2 -> Write/Action
  Write/1(WriteCMD) -> Merge/2
  If/1 -> Reset/Action
  Detect Increase/1 -> OR/1
  AND/1 -> [VTQD_WriteComboCMD_flg]  "VTQD_WriteComboCMD_flg"
  [VTQD_ComboKeyCMD_enum] -> Write/1(Input)
  [VTQD_ComboKeyCMD_enum] -> Detect Change/1
  [VTQD_ResetComboKey_flg] -> If/1
  [VTQD_ComboKeyEn_flg] -> Detect Increase/1
  Detect Change/1 -> AND/1
  Maintain/1(KeepKey2) -> Merge/3
  Constant4/1 -> Equal1/2
  If/3 -> Maintain/Action
  Delay/1 -> Equal2/1
  Merge/1 -> Data Type Conversion/1
  Reset/1(ResetToZero) -> Merge/1
  Equal2/1 -> AND/3
  Constant2/1 -> Equal2/2
  Equal1/1 -> AND/2
  [VTQD_ComboKey1_enum] -> Delay/1
  [VTQD_ComboKeyReset_flg] -> OR/2
  [VTQD_ComboKeyCMD_enum] -> Equal1/1
  [VTQD_WriteComboCMD_flg] -> If/2
  OR/1 -> [VTQD_ResetComboKey_flg]  "VTQD_ResetComboKey_flg"
  VTQD_ComboKey1_enum/1 -> [VTQD_ComboKey1_enum]
  [VTQD_ComboKey2_enum] -> Delay1/1
  Constant3/1 -> Equal3/2
  Delay1/1 -> Equal3/1
  Equal3/1 -> AND/4
  Delay2/1 -> Maintain/1(Input)
  [VTQD_ComboKey2_enum] -> Delay2/1
  Data Type Conversion/1 -> [VTQD_ComboKey2_enum]  "VTQD_Function3Off2_enum"

== system tqd/TQD/Input_Convert/Input Signal Convert/Big Mike Combo V2 /Combo Key Detection/Function3/Key3 ==
  VTQD_ComboKeyCMD_enum : Inport
  VTQD_ComboKeyEn_flg : Inport  Port=2
  VTQD_ComboKeyReset_flg : Inport  Port=3
  VTQD_ComboKey2_enum : Inport  Port=4
  AND : Logic  Inputs=4  AllPortsSameDT=off  OutDataTypeStr=boolean
  Constant1 : Constant  Value=KTQD_Function3Off3_enum
  Constant2 : Constant  Value=ENUM_COMBOKEY_NONE
  Constant3 : Constant  Value=ENUM_COMBOKEY_NONE
  Constant4 : Constant  Value=ENUM_COMBOKEY_NONE
  Data Type Conversion : DataTypeConversion  OutDataTypeStr=uint8
  Delay : Delay  DelayLength=1  InitialCondition=uint8(0)
      settings: AttributesFormatString=%<InitialCondition>
  Delay1 : Delay  DelayLength=1  InitialCondition=uint8(0)
      settings: AttributesFormatString=%<InitialCondition>
  Delay2 : Delay  DelayLength=1  InitialCondition=uint8(0)
      settings: AttributesFormatString=%<InitialCondition>
  Detect Change : simulink/Logic and Bit Operations/Detect Change  vinit=boolean(0)  OutDataTypeStr=boolean
  Detect Increase : simulink/Logic and Bit Operations/Detect Increase  vinit=boolean(0)  OutDataTypeStr=boolean
  Equal : RelationalOperator  Operator===  OutDataTypeStr=boolean  RndMeth=Simplest
  Equal1 : RelationalOperator  Operator=~=  OutDataTypeStr=boolean  RndMeth=Simplest
  Equal2 : RelationalOperator  Operator=~=  OutDataTypeStr=boolean  RndMeth=Simplest
  Equal3 : RelationalOperator  Operator===  OutDataTypeStr=boolean  RndMeth=Simplest
  If : If  NumInputs=2  IfExpression=u1 ~=0  ElseIfExpressions=u2 ~= 0
  Maintain : Subsystem  TreatAsAtomicUnit=on
  Merge : Merge  Inputs=3
  OR : Logic  Operator=OR  AllPortsSameDT=off  OutDataTypeStr=boolean
  Reset : Subsystem  TreatAsAtomicUnit=on
  Write : Subsystem  TreatAsAtomicUnit=on
  VTQD_ComboKey3_enum : Outport
  VTQD_Key3Pass_flg : Outport  Port=2
  wires:
  VTQD_ComboKey2_enum/1 -> [VTQD_ComboKey2_enum]
  OR/1 -> [VTQD_ResetComboKey_flg]  "VTQD_ResetComboKey_flg"
  [VTQD_WriteComboCMD_flg] -> If/2
  [VTQD_ComboKeyCMD_enum] -> Equal1/1
  [VTQD_ComboKeyReset_flg] -> OR/2
  [VTQD_ComboKey2_enum] -> Delay/1
  Equal1/1 -> AND/2
  Constant2/1 -> Equal2/2
  Equal2/1 -> AND/3
  Reset/1(ResetToZero) -> Merge/1
  Merge/1 -> Data Type Conversion/1
  Delay/1 -> Equal2/1
  If/3 -> Maintain/Action
  Constant4/1 -> Equal1/2
  Maintain/1(KeepKey3) -> Merge/3
  Detect Change/1 -> AND/1
  [VTQD_ComboKeyEn_flg] -> Detect Increase/1
  [VTQD_ResetComboKey_flg] -> If/1
  [VTQD_ComboKeyCMD_enum] -> Detect Change/1
  [VTQD_ComboKeyCMD_enum] -> Write/1(Input)
  AND/1 -> [VTQD_WriteComboCMD_flg]  "VTQD_WriteComboCMD_flg"
  Detect Increase/1 -> OR/1
  If/1 -> Reset/Action
  Write/1(WriteCMD) -> Merge/2
  If/2 -> Write/Action
  Constant1/1 -> Equal/2
  Equal/1 -> [VTQD_Key3Pass_flg]  "VTQD_Function3Off3Pass_flg"
  VTQD_ComboKeyCMD_enum/1 -> [VTQD_ComboKeyCMD_enum]
  VTQD_ComboKeyReset_flg/1 -> [VTQD_ComboKeyReset_flg]
  VTQD_ComboKeyEn_flg/1 -> [VTQD_ComboKeyEn_flg]
  [VTQD_ComboKey3_enum] -> VTQD_ComboKey3_enum/1
  [VTQD_ComboKey3_enum] -> Equal/1
  [VTQD_Key3Pass_flg] -> VTQD_Key3Pass_flg/1
  Delay1/1 -> Equal3/1
  Equal3/1 -> AND/4
  Constant3/1 -> Equal3/2
  [VTQD_ComboKey3_enum] -> Delay1/1
  Delay2/1 -> Maintain/1(Input)
  [VTQD_ComboKey3_enum] -> Delay2/1
  Data Type Conversion/1 -> [VTQD_ComboKey3_enum]  "VTQD_Function3Off3_enum"

== system tqd/TQD/Input_Convert/Input Signal Convert/Big Mike Combo V2 /Combo Key Detection/Function3/Key4 ==
  VTQD_ComboKeyCMD_enum : Inport
  VTQD_ComboKeyEn_flg : Inport  Port=2
  VTQD_ComboKeyReset_flg : Inport  Port=3
  VTQD_ComboKey3_enum : Inport  Port=4
  AND : Logic  Inputs=4  AllPortsSameDT=off  OutDataTypeStr=boolean
  Constant1 : Constant  Value=KTQD_Function3Off4_enum
  Constant2 : Constant  Value=ENUM_COMBOKEY_NONE
  Constant3 : Constant  Value=ENUM_COMBOKEY_NONE
  Constant4 : Constant  Value=ENUM_COMBOKEY_NONE
  Data Type Conversion : DataTypeConversion  OutDataTypeStr=uint8
  Delay : Delay  DelayLength=1  InitialCondition=uint8(0)
      settings: AttributesFormatString=%<InitialCondition>
  Delay1 : Delay  DelayLength=1  InitialCondition=uint8(0)
      settings: AttributesFormatString=%<InitialCondition>
  Delay2 : Delay  DelayLength=1  InitialCondition=uint8(0)
      settings: AttributesFormatString=%<InitialCondition>
  Detect Change : simulink/Logic and Bit Operations/Detect Change  vinit=boolean(0)  OutDataTypeStr=boolean
  Detect Increase : simulink/Logic and Bit Operations/Detect Increase  vinit=boolean(0)  OutDataTypeStr=boolean
  Equal : RelationalOperator  Operator===  OutDataTypeStr=boolean  RndMeth=Simplest
  Equal1 : RelationalOperator  Operator=~=  OutDataTypeStr=boolean  RndMeth=Simplest
  Equal2 : RelationalOperator  Operator=~=  OutDataTypeStr=boolean  RndMeth=Simplest
  Equal3 : RelationalOperator  Operator===  OutDataTypeStr=boolean  RndMeth=Simplest
  If : If  NumInputs=2  IfExpression=u1 ~=0  ElseIfExpressions=u2 ~= 0
  Maintain : Subsystem  TreatAsAtomicUnit=on
  Merge : Merge  Inputs=3
  OR : Logic  Operator=OR  AllPortsSameDT=off  OutDataTypeStr=boolean
  Reset : Subsystem  TreatAsAtomicUnit=on
  Write : Subsystem  TreatAsAtomicUnit=on
  VTQD_ComboKey4_enum : Outport
  VTQD_Key4Pass_flg : Outport  Port=2
  wires:
  [VTQD_ComboKey4_enum] -> Equal/1
  VTQD_ComboKeyEn_flg/1 -> [VTQD_ComboKeyEn_flg]
  VTQD_ComboKeyReset_flg/1 -> [VTQD_ComboKeyReset_flg]
  VTQD_ComboKeyCMD_enum/1 -> [VTQD_ComboKeyCMD_enum]
  Equal/1 -> [VTQD_Key4Pass_flg]  "VTQD_Function3Off4Pass_flg"
  Constant1/1 -> Equal/2
  If/2 -> Write/Action
  Write/1(WriteCMD) -> Merge/2
  If/1 -> Reset/Action
  Detect Increase/1 -> OR/1
  AND/1 -> [VTQD_WriteComboCMD_flg]  "VTQD_WriteComboCMD_flg"
  [VTQD_ComboKeyCMD_enum] -> Write/1(Input)
  [VTQD_ComboKeyCMD_enum] -> Detect Change/1
  [VTQD_ResetComboKey_flg] -> If/1
  [VTQD_ComboKeyEn_flg] -> Detect Increase/1
  Detect Change/1 -> AND/1
  Maintain/1(KeepKey4) -> Merge/3
  Constant4/1 -> Equal1/2
  If/3 -> Maintain/Action
  Delay/1 -> Equal2/1
  Merge/1 -> Data Type Conversion/1
  Reset/1(ResetToZero) -> Merge/1
  Equal2/1 -> AND/3
  Constant2/1 -> Equal2/2
  Equal1/1 -> AND/2
  [VTQD_ComboKey3_enum] -> Delay/1
  [VTQD_ComboKeyReset_flg] -> OR/2
  [VTQD_ComboKeyCMD_enum] -> Equal1/1
  [VTQD_WriteComboCMD_flg] -> If/2
  OR/1 -> [VTQD_ResetComboKey_flg]  "VTQD_ResetComboKey_flg"
  VTQD_ComboKey3_enum/1 -> [VTQD_ComboKey3_enum]
  [VTQD_ComboKey4_enum] -> Delay1/1
  Constant3/1 -> Equal3/2
  Delay1/1 -> Equal3/1
  Equal3/1 -> AND/4
  [VTQD_Key4Pass_flg] -> VTQD_Key4Pass_flg/1
  [VTQD_ComboKey4_enum] -> VTQD_ComboKey4_enum/1
  [VTQD_ComboKey4_enum] -> Delay2/1
  Delay2/1 -> Maintain/1(Input)
  Data Type Conversion/1 -> [VTQD_ComboKey4_enum]  "VTQD_Function3Off4_enum"

== system tqd/TQD/Input_Convert/Input Signal Convert/Big Mike Combo V2 /Combo Key Detection/Function3/Key5 ==
  VTQD_ComboKeyCMD_enum : Inport
  VTQD_ComboKeyEn_flg : Inport  Port=2
  VTQD_ComboKeyReset_flg : Inport  Port=3
  VTQD_ComboKey4_enum : Inport  Port=4
  AND : Logic  Inputs=4  AllPortsSameDT=off  OutDataTypeStr=boolean
  Constant1 : Constant  Value=KTQD_Function3Off5_enum
  Constant2 : Constant  Value=ENUM_COMBOKEY_NONE
  Constant3 : Constant  Value=ENUM_COMBOKEY_NONE
  Constant4 : Constant  Value=ENUM_COMBOKEY_NONE
  Data Type Conversion : DataTypeConversion  OutDataTypeStr=uint8
  Delay : Delay  DelayLength=1  InitialCondition=uint8(0)
      settings: AttributesFormatString=%<InitialCondition>
  Delay1 : Delay  DelayLength=1  InitialCondition=uint8(0)
      settings: AttributesFormatString=%<InitialCondition>
  Delay2 : Delay  DelayLength=1  InitialCondition=uint8(0)
      settings: AttributesFormatString=%<InitialCondition>
  Detect Change : simulink/Logic and Bit Operations/Detect Change  vinit=boolean(0)  OutDataTypeStr=boolean
  Detect Increase : simulink/Logic and Bit Operations/Detect Increase  vinit=boolean(0)  OutDataTypeStr=boolean
  Equal : RelationalOperator  Operator===  OutDataTypeStr=boolean  RndMeth=Simplest
  Equal1 : RelationalOperator  Operator=~=  OutDataTypeStr=boolean  RndMeth=Simplest
  Equal2 : RelationalOperator  Operator=~=  OutDataTypeStr=boolean  RndMeth=Simplest
  Equal3 : RelationalOperator  Operator===  OutDataTypeStr=boolean  RndMeth=Simplest
  If : If  NumInputs=2  IfExpression=u1 ~=0  ElseIfExpressions=u2 ~= 0
  Maintain : Subsystem  TreatAsAtomicUnit=on
  Merge : Merge  Inputs=3
  OR : Logic  Operator=OR  AllPortsSameDT=off  OutDataTypeStr=boolean
  Reset : Subsystem  TreatAsAtomicUnit=on
  Write : Subsystem  TreatAsAtomicUnit=on
  VTQD_ComboKey5_enum : Outport
  VTQD_Key5Pass_flg : Outport  Port=2
  wires:
  [VTQD_Key5Pass_flg] -> VTQD_Key5Pass_flg/1
  Equal3/1 -> AND/4
  Delay1/1 -> Equal3/1
  Constant3/1 -> Equal3/2
  [VTQD_ComboKey5_enum] -> Delay1/1
  VTQD_ComboKey4_enum/1 -> [VTQD_ComboKey4_enum]
  OR/1 -> [VTQD_ResetComboKey_flg]  "VTQD_ResetComboKey_flg"
  [VTQD_WriteComboCMD_flg] -> If/2
  [VTQD_ComboKeyCMD_enum] -> Equal1/1
  [VTQD_ComboKeyReset_flg] -> OR/2
  [VTQD_ComboKey4_enum] -> Delay/1
  Equal1/1 -> AND/2
  Constant2/1 -> Equal2/2
  Equal2/1 -> AND/3
  Reset/1(ResetToZero) -> Merge/1
  Merge/1 -> Data Type Conversion/1
  Delay/1 -> Equal2/1
  If/3 -> Maintain/Action
  Constant4/1 -> Equal1/2
  Maintain/1(KeepKey5) -> Merge/3
  Detect Change/1 -> AND/1
  [VTQD_ComboKeyEn_flg] -> Detect Increase/1
  [VTQD_ResetComboKey_flg] -> If/1
  [VTQD_ComboKeyCMD_enum] -> Detect Change/1
  [VTQD_ComboKeyCMD_enum] -> Write/1(Input)
  AND/1 -> [VTQD_WriteComboCMD_flg]  "VTQD_WriteComboCMD_flg"
  Detect Increase/1 -> OR/1
  If/1 -> Reset/Action
  Write/1(WriteCMD) -> Merge/2
  If/2 -> Write/Action
  Constant1/1 -> Equal/2
  Equal/1 -> [VTQD_Key5Pass_flg]  "VTQD_Function3Off5Pass_flg"
  VTQD_ComboKeyCMD_enum/1 -> [VTQD_ComboKeyCMD_enum]
  VTQD_ComboKeyReset_flg/1 -> [VTQD_ComboKeyReset_flg]
  VTQD_ComboKeyEn_flg/1 -> [VTQD_ComboKeyEn_flg]
  [VTQD_ComboKey5_enum] -> Equal/1
  [VTQD_ComboKey5_enum] -> VTQD_ComboKey5_enum/1
  [VTQD_ComboKey5_enum] -> Delay2/1
  Delay2/1 -> Maintain/1(Input)
  Data Type Conversion/1 -> [VTQD_ComboKey5_enum]  "VTQD_Function3Off5_enum"
